simulink model "gm_max_frequency_reduced"  (R2020a)
settings: Solver=FixedStepDiscrete  StartTime=0.0  StopTime=1e-2  RelTol=1e-3
model workspace (MAT data in the model file):
  amplitud = 2047
  fft_length = 16
  samples_per_period = 3
  sampling_time = 1e-06
libraries: dspsrcs4 x1, dsphdlxfrm x1, hdlsllib x1
settings Model: Creator=giova  LastModifiedBy=giova
settings SolverCC: AutoInsertRateTranBlk=on
settings DataIOCC: SaveOutput=off  SaveTime=off
settings OptimizationCC: BlockReduction=off  ConditionallyExecuteInputs=off  DefaultParameterBehavior=Inlined
settings DebuggingCC: AlgebraicLoopMsg=error  InheritedTsInSrcMsg=none  SingleTaskRateTransMsg=error  StrictBusMsg=ErrorOnBusTreatedAsVector  ArithmeticOperatorsInVariantConditions=warning
settings HardwareCC: ProdBitPerPointer=32  ProdBitPerSizeT=32  ProdBitPerPtrDiffT=32  ProdLargestAtomicFloat=None  ProdIntDivRoundTo=Undefined  ProdEndianess=Unspecified  ProdWordSize=32  ProdHWDeviceType=ASIC/FPGA->ASIC/FPGA  TargetBitPerPointer=64  TargetBitPerSizeT=64  TargetBitPerPtrDiffT=64  TargetLongLongMode=on  TargetIntDivRoundTo=Zero  TargetEndianess=LittleEndian  TargetWordSize=64  TargetHWDeviceType=Custom Processor->MATLAB Host Computer  ProdEqTarget=off
settings SFSimCC: SimUseLocalCustomCode=off  CustomCodeUndefinedFunction=UseInterfaceOnly
settings RTWCC: RTWUseLocalCustomCode=off
settings CodeAppCC: StateflowObjectComments=on
settings GRTTargetCC: TargetLangStandard=C89/C90 (ANSI)

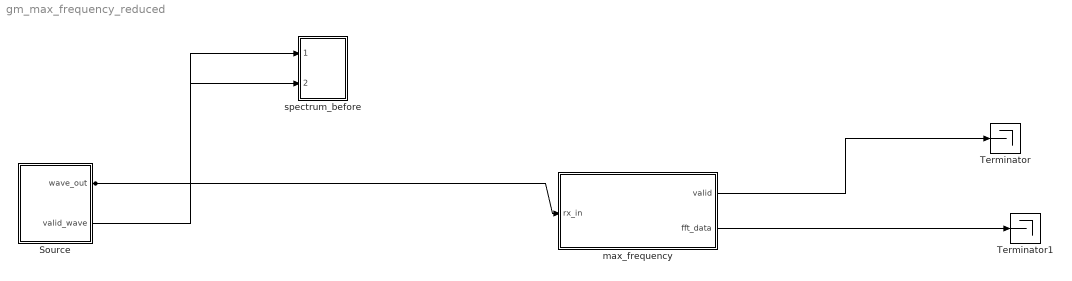
== system gm_max_frequency_reduced ==
  Source : Subsystem
  Terminator : Terminator
  Terminator1 : Terminator
  max_frequency : Subsystem
  spectrum_before : Subsystem
  wires:
  max_frequency/1(valid) -> Terminator/1
  max_frequency/2(fft_data) -> Terminator1/1
  Source/2(valid_wave) -> spectrum_before/2(valid_wave)
  Source/1(wave_out) -> max_frequency/1(rx_in), spectrum_before/1(wave_out)

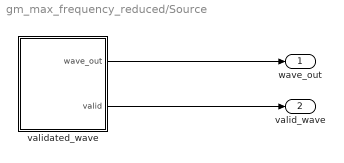
== system gm_max_frequency_reduced/Source ==
  validated_wave : Subsystem
  wave_out : Outport  VectorParamsAs1DForOutWhenUnconnected=off
  valid_wave : Outport  Port=2  VectorParamsAs1DForOutWhenUnconnected=off
  wires:
  validated_wave/1(wave_out) -> wave_out/1
  validated_wave/2(valid) -> valid_wave/1

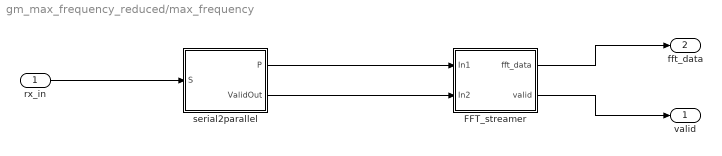
== system gm_max_frequency_reduced/max_frequency ==
  rx_in : Inport  OutDataTypeStr=fixdt(1, 12, 0)  PortDimensions=1  SampleTime=1e-06
      settings: SignalType=complex
  FFT_streamer : Subsystem
  serial2parallel : Subsystem
  valid : Outport
  fft_data : Outport  Port=2
  wires:
  rx_in/1 -> serial2parallel/1(S)
  FFT_streamer/1(fft_data) -> fft_data/1
  FFT_streamer/2(valid) -> valid/1
  serial2parallel/1(P) -> FFT_streamer/1(In1)
  serial2parallel/2(ValidOut) -> FFT_streamer/2(In2)

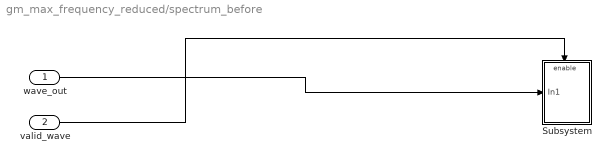
== system gm_max_frequency_reduced/spectrum_before ==
  wave_out : Inport
  valid_wave : Inport  Port=2
  Subsystem : Subsystem
  wires:
  valid_wave/1 -> Subsystem/Enable
  wave_out/1 -> Subsystem/1(In1)

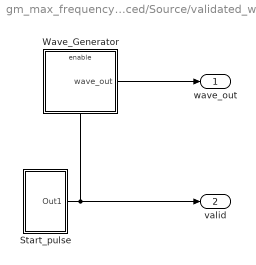
== system gm_max_frequency_reduced/Source/validated_wave ==
  Start_pulse : Subsystem
  Wave_Generator : Subsystem
  wave_out : Outport  VectorParamsAs1DForOutWhenUnconnected=off
  valid : Outport  Port=2  VectorParamsAs1DForOutWhenUnconnected=off
  wires:
  Wave_Generator/1(wave_out) -> wave_out/1
  Start_pulse/1(Out1) -> Wave_Generator/Enable, valid/1

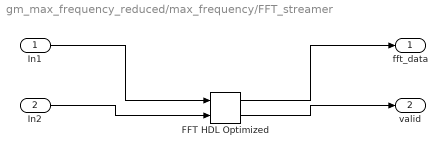
== system gm_max_frequency_reduced/max_frequency/FFT_streamer ==
  In1 : Inport  OutDataTypeStr=fixdt(1, 12, 0)  PortDimensions=[16]  SampleTime=1.6e-05
      settings: SignalType=complex
  In2 : Inport  Port=2  OutDataTypeStr=boolean  PortDimensions=1  SampleTime=1.6e-05
  FFT HDL Optimized : dsphdlxfrm/FFT HDL Optimized  FFTLength=fft_length  Architecture=Streaming Radix 2^2  ComplexMultiplication=Use 4 multipliers and 2 adders  BitReversedOutput=off  BitReversedInput=off  Normalize=on  SimulateUsing=Code generation  RoundingMethod=Floor  ResetInputPort=off  StartOutputPort=off  EndOutputPort=off
      settings: SourceProductBaseCode=DS
  fft_data : Outport
  valid : Outport  Port=2
  wires:
  In1/1 -> FFT HDL Optimized/1
  In2/1 -> FFT HDL Optimized/2
  FFT HDL Optimized/1 -> fft_data/1
  FFT HDL Optimized/2 -> valid/1

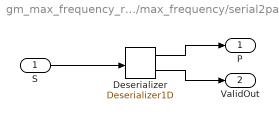
== system gm_max_frequency_reduced/max_frequency/serial2parallel ==
  S : Inport  OutDataTypeStr=fixdt(1, 12, 0)  PortDimensions=1  SampleTime=1e-06
      settings: SignalType=complex
  Deserializer : hdlsllib/HDL Operations/Deserializer1D  Ratio=16  IdleCycles=0  InitialCondition="fi(0,1,12,0,\"hex\",\"000 + 000 i\")"  startIn=off  validIn=off  validOut=on  inputDataDimensions=1  inputSampleTime=1e-06  inputSignalType=complex
      settings: SourceProductBaseCode=SL
  P : Outport
  ValidOut : Outport  Port=2
  wires:
  S/1 -> Deserializer/1
  Deserializer/1 -> P/1
  Deserializer/2 -> ValidOut/1

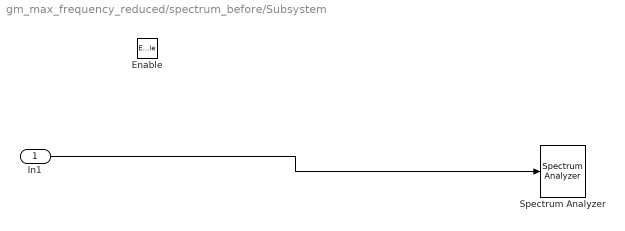
== system gm_max_frequency_reduced/spectrum_before/Subsystem ==
  In1 : Inport
  Enable : EnablePort
  Spectrum Analyzer : SpectrumAnalyzer
  wires:
  In1/1 -> Spectrum Analyzer/1

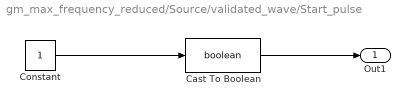
== system gm_max_frequency_reduced/Source/validated_wave/Start_pulse ==
  Cast To Boolean : DataTypeConversion  OutDataTypeStr=boolean
  Constant : Constant  SampleTime=sampling_time  LockScale=on
  Out1 : Outport  VectorParamsAs1DForOutWhenUnconnected=off
  wires:
  Constant/1 -> Cast To Boolean/1
  Cast To Boolean/1 -> Out1/1

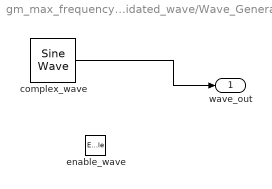
== system gm_max_frequency_reduced/Source/validated_wave/Wave_Generator ==
  enable_wave : EnablePort
  complex_wave : dspsrcs4/Sine Wave  Amplitude=amplitud  Frequency=1/(sampling_time*samples_per_period)  Phase=0  SampleMode=Discrete  OutComplex=Complex  CompMethod=Table lookup  TableSize=Speed  SampleTime=sampling_time  SamplesPerFrame=1  ResetState=Restart at time zero  OutputFrames=off  dataType=Fixed-point  wordLen=12  udDataType=sfix(16)  fracBitsMode=User-defined  numFracBits=0  OutDataTypeStr=fixdt(1,12,0)  LastOutDataTypeStr=fixdt(1,12,0)
  wave_out : Outport  InitialOutput=0  VectorParamsAs1DForOutWhenUnconnected=off
  wires:
  complex_wave/1 -> wave_out/1
